simulink model "FullDimStateWatcher"  (R2018b)
settings: Solver=VariableStepAuto  StartTime=0.0  StopTime=80  RelTol=1e-3  EnableMultiTasking=on
settings Model: Creator=B303  LastModifiedBy=erange
settings DataIOCC: LimitDataPoints=on
settings OptimizationCC: LifeSpan=inf
settings DebuggingCC: AllowSymbolicDim=off  SFUnexpectedBacktrackingDiag=warning  SFNoUnconditionalDefaultTransitionDiag=warning  SFExecutionAtInitializationDiag=none
settings ModelReferenceCC: PropagateSignalLabelsOutOfModel=off
settings SFSimCC: SimUseLocalCustomCode=off
settings RTWCC: RTWUseLocalCustomCode=off
settings CodeAppCC: StateflowObjectComments=on
settings GRTTargetCC: TargetLangStandard=C89/C90 (ANSI)
settings ConfigComp: CovMetricSettings=dw  CovHtmlReporting=on  CovSaveCumulativeToWorkspaceVar=on  CovSaveSingleToWorkspaceVar=on  CovExternalEMLEnable=off

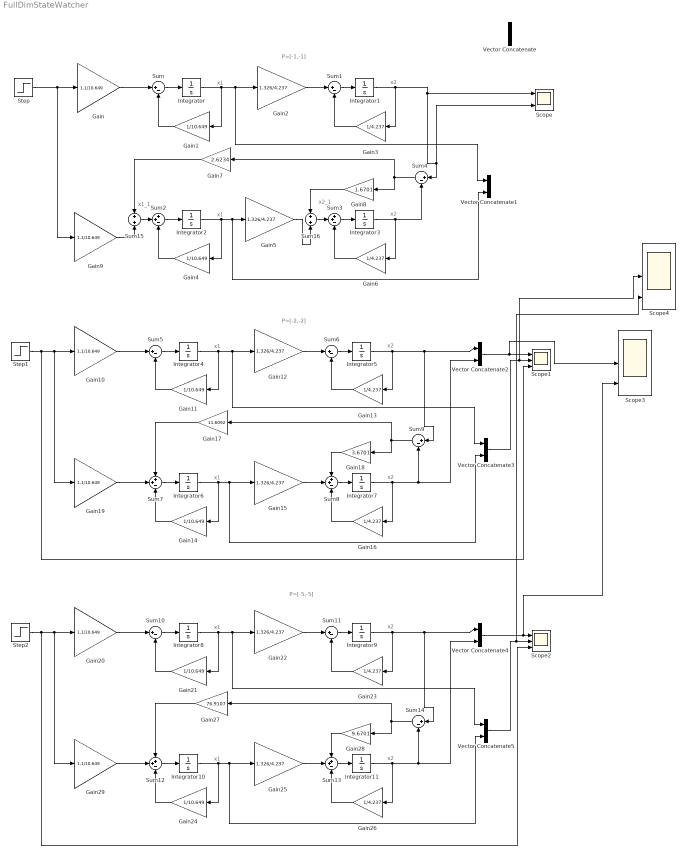
== system FullDimStateWatcher ==
  note: x2_1
  note: x1_1
  note: P=[-5,-5]
  note: x1
  note: x2
  note: x2
  note: x1
  note: x2
  note: x2
  note: x1
  note: x1
  note: x2
  note: x2
  note: x1
  note: x1
  note: P=[-2,-2]
  note: P=[-1,-1]
  Gain{,9..10,19..20,29} (6 alike) : Gain  Gain=1.1/10.649
  Gain{1,4,11,14,21,24} (6 alike) : Gain  Gain=1/10.649
  Gain{2,5,12,15,22,25} (6 alike) : Gain  Gain=1.326/4.237
  Gain{3,6,13,16,23,26} (6 alike) : Gain  Gain=1/4.237
  Gain17 : Gain  Gain=11.6092
  Gain18 : Gain  Gain=3.6701
  Gain27 : Gain  Gain=76.9107
  Gain28 : Gain  Gain=9.6701
  Gain7 : Gain  Gain=2.6234
  Gain8 : Gain  Gain=1.6701
  Integrator{,1..3,6..7,10..11} (8 alike) : Integrator
  Integrator4 : Integrator  InitialCondition=2
  Integrator5 : Integrator  InitialCondition=5
  Integrator8 : Integrator  InitialCondition=2
  Integrator9 : Integrator  InitialCondition=5
  Scope : Scope  NumInputPorts=2
  Scope{1..4} (4 alike) : Scope  NumInputPorts=3
  Step : Step  Time=0  SampleTime=0
  Step1 : Step  Time=0  After=3  SampleTime=0
  Step2 : Step  Time=0  After=3  SampleTime=0
  Sum{,1,4..6,9..11,14} (9 alike) : Sum  Inputs=|+-
  Sum{2..3,7..8,12..13} (6 alike) : Sum  Inputs=++-
  Sum15 : Sum
  Sum16 : Sum
  Vector Concatenate{,1..5} (6 alike) : Concatenate  Mode=Multidimensional array  ConcatenateDimension=2
  wires:
  Sum/1 -> Integrator/1
  Gain/1 -> Sum/1
  Integrator/1 -> Gain1/1, Vector Concatenate1/1, Gain2/1
  Gain1/1 -> Sum/2
  Gain2/1 -> Sum1/1
  Sum1/1 -> Integrator1/1
  Integrator1/1 -> Gain3/1, Scope/1, Sum4/1, Scope/2
  Gain3/1 -> Sum1/2
  Step/1 -> Gain9/1, Gain/1
  Sum3/1 -> Integrator3/1
  Integrator3/1 -> Sum4/2, Gain6/1
  Integrator2/1 -> Gain4/1, Vector Concatenate1/2, Gain5/1
  Sum2/1 -> Integrator2/1
  Sum4/1 -> Gain7/1, Gain8/1
  Gain6/1 -> Sum3/3
  Gain4/1 -> Sum2/3
  Gain19/1 -> Sum7/2
  Gain15/1 -> Sum8/2
  Gain16/1 -> Sum8/3
  Gain14/1 -> Sum7/3
  Gain12/1 -> Sum6/1
  Step1/1 -> Scope1/3, Gain19/1, Gain10/1
  Integrator5/1 -> Gain13/1, Vector Concatenate2/1, Sum9/1
  Gain10/1 -> Sum5/1
  Gain13/1 -> Sum6/2
  Integrator4/1 -> Gain11/1, Vector Concatenate3/1, Gain12/1
  Sum5/1 -> Integrator4/1
  Sum7/1 -> Integrator6/1
  Integrator6/1 -> Gain14/1, Vector Concatenate3/2, Gain15/1
  Vector Concatenate2/1 -> Scope3/2, Scope1/1
  Sum8/1 -> Integrator7/1
  Sum6/1 -> Integrator5/1
  Integrator7/1 -> Vector Concatenate2/2, Sum9/2, Gain16/1
  Gain11/1 -> Sum5/2
  Vector Concatenate3/1 -> Scope4/2, Scope1/2
  Gain18/1 -> Sum8/1
  Sum9/1 -> Gain17/1, Gain18/1
  Gain17/1 -> Sum7/1
  Gain29/1 -> Sum12/2
  Gain25/1 -> Sum13/2
  Gain26/1 -> Sum13/3
  Gain24/1 -> Sum12/3
  Gain22/1 -> Sum11/1
  Step2/1 -> Scope2/3, Gain29/1, Gain20/1
  Integrator9/1 -> Gain23/1, Vector Concatenate4/1, Sum14/1
  Gain20/1 -> Sum10/1
  Gain23/1 -> Sum11/2
  Integrator8/1 -> Gain21/1, Vector Concatenate5/1, Gain22/1
  Sum10/1 -> Integrator8/1
  Sum12/1 -> Integrator10/1
  Integrator10/1 -> Gain24/1, Vector Concatenate5/2, Gain25/1
  Vector Concatenate4/1 -> Scope3/3, Scope2/1
  Sum13/1 -> Integrator11/1
  Sum11/1 -> Integrator9/1
  Integrator11/1 -> Vector Concatenate4/2, Sum14/2, Gain26/1
  Gain21/1 -> Sum10/2
  Vector Concatenate5/1 -> Scope4/3, Scope2/2
  Gain28/1 -> Sum13/1
  Sum14/1 -> Gain27/1, Gain28/1
  Gain27/1 -> Sum12/1
  Sum15/1 -> Sum2/2
  Gain9/1 -> Sum15/2
  Gain7/1 -> Sum15/1
  Sum16/1 -> Sum3/2
  Gain5/1 -> Sum16/2
  Gain8/1 -> Sum16/1
